simulink model "PID"  (R2017a)
settings: Solver=ode45  StartTime=0.0  StopTime=50  RelTol=1e-3  EnableMultiTasking=on
undefined symbols (not defined in the file): PID, thesis_lib
libraries: realtime_pacer_lib x1
settings Model: Creator=Waleed Niaz  LastModifiedBy=Waleed Niaz
settings DataIOCC: LimitDataPoints=on  SaveFormat=Array  SignalLoggingSaveFormat=ModelDataLogs
settings OptimizationCC: BooleanDataType=off
settings DebuggingCC: SaveWithParameterizedLinksMsg=none  UnderspecifiedInitializationDetection=Classic  MergeDetectMultiDrivingBlocksExec=none  SignalResolutionControl=TryResolveAllWithWarning  MultiTaskDSMMsg=warning  MultiTaskCondExecSysMsg=none
settings HardwareCC: TargetUnknown=on
settings ModelReferenceCC: PropagateSignalLabelsOutOfModel=off
settings GRTTargetCC: TargetLangStandard=C89/C90 (ANSI)  CombineOutputUpdateFcns=off  GRTInterface=on
settings ConfigComp: CovMetricSettings=dw  CovHtmlReporting=on  CovSaveCumulativeToWorkspaceVar=on  CovSaveSingleToWorkspaceVar=on  CovExternalEMLEnable=off

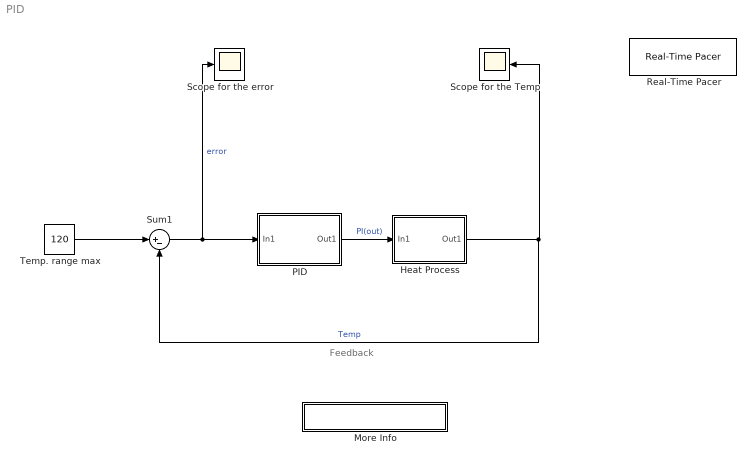
== system PID ==
  note: Feedback
  Heat Process : Subsystem  mask(Process){T2=120, T1=75, F1=4, V=6}
      mask prompts: T2 "Temperature of hot water"; T1 "Temperature of cold water"; F1 "Flow rate of cold water"; V "Volume of the tank"
      mask help: The values for the temperature should be expressed in either degree Rankine or Kelvin.
      mask Display: disp('PROCESS')
  More Info : Subsystem
      mask Display: disp('Click here more information')
  PID : Subsystem  AncestorBlock=thesis_lib/PID  mask(PID Controller (Zervin's block)){P=0.9, I=0.4, D=0}
      mask prompts: P "Proportional Gain, Kp"; I "Integral Gain, Ki"; D "Derivative Gain, Kd"
      mask help: This Block is a model of a PID controller
      mask Help: Enter a value for Kp, Ki, and Kd.
      mask Display:
      | disp('PID \n\n');
      | disp('Controller');
  Real-Time Pacer : realtime_pacer_lib/Real-Time Pacer  simTimePerRealTime=1
  Scope for the Temp : Scope
  Scope for the error : Scope
  Sum1 : Sum  Inputs=|+-
  Temp. range max : Constant  Value=120  VectorParams1D=off
  wires:
  Sum1/1 -> Scope for the error/1, PID/1(In1)  "error"
  PID/1(Out1) -> Heat Process/1(In1)  "PI(out)"
  Heat Process/1(Out1) -> Sum1/2, Scope for the Temp/1  "Temp"
  Temp. range max/1 -> Sum1/1

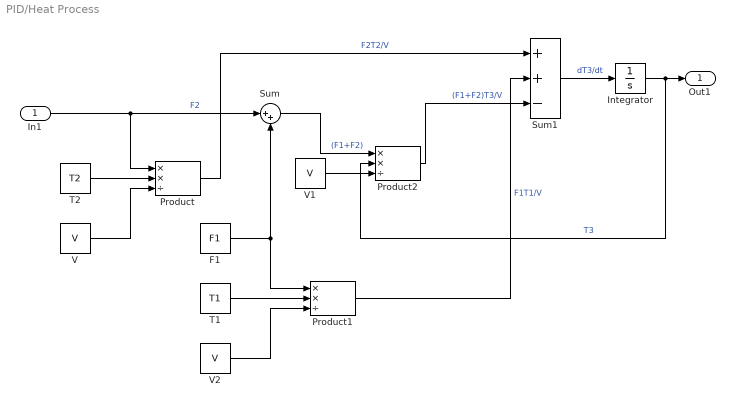
== system PID/Heat Process ==
  In1 : Inport
  F1 : Constant  Value=F1
  Integrator : Integrator  InitialCondition=T1
  Product : Product  Inputs=**/  SaturateOnIntegerOverflow=on  RndMeth=Zero  InputSameDT=on  OutDataTypeStr=Inherit: Same as first input
  Product1 : Product  Inputs=**/  SaturateOnIntegerOverflow=on  RndMeth=Zero  InputSameDT=on  OutDataTypeStr=Inherit: Same as first input
  Product2 : Product  Inputs=**/  SaturateOnIntegerOverflow=on  RndMeth=Zero  InputSameDT=on  OutDataTypeStr=Inherit: Same as first input
  Sum : Sum  Inputs=|++  SaturateOnIntegerOverflow=on  InputSameDT=on  OutDataTypeStr=Inherit: Same as first input
  Sum1 : Sum  Inputs=|++-  SaturateOnIntegerOverflow=on  InputSameDT=on  OutDataTypeStr=Inherit: Same as first input
  T1 : Constant  Value=T1
  T2 : Constant  Value=T2
  V : Constant  Value=V
  V1 : Constant  Value=V
  V2 : Constant  Value=V
  Out1 : Outport
  wires:
  In1/1 -> Product/1, Sum/1  "F2"
  V/1 -> Product/3
  F1/1 -> Product1/1, Sum/2
  T1/1 -> Product1/2
  V2/1 -> Product1/3
  V1/1 -> Product2/3
  Sum/1 -> Product2/1  "(F1+F2)"
  Product/1 -> Sum1/1  "F2T2/V"
  Product1/1 -> Sum1/2  "F1T1/V"
  Product2/1 -> Sum1/3  "(F1+F2)T3/V"
  Sum1/1 -> Integrator/1  "dT3/dt"
  Integrator/1 -> Product2/2, Out1/1  "T3"
  T2/1 -> Product/2

== system PID/More Info ==
  note: Before starting the simulation of the
      | system, the constant parameters of the system
      | must first be supplied to the model.
      | i.e the PI constant values
  note: Here are the parameters that needs to be specified:
  note: 1.) For the Temp. set point block, the Temperature set point or the desired
      | temperature.
      | 2.) For the PID controller block, the value of Kp, Ki and Kd.
      | 3.) For the process block, the Temperature of the incoming flows, the flowrate of the cold water and the volume of the tank.
      | 4.) Real time pacer uses the matlab pause and show the real time simulation in seconds.
      | 5.) Real time pacer library is not a built-in library we have to download it online.
      | 6.) If real time pacer block is not found then run again the file real_time_pacer.lib and add the block.
  note: The response or the result of the simulation can be viewed
      | by double-clicking the scope blocks.

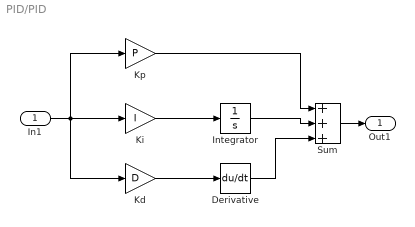
== system PID/PID ==
  In1 : Inport
  Derivative : Derivative
  Integrator : Integrator
  Kd : Gain  Gain=D  SaturateOnIntegerOverflow=on  OutDataTypeStr=Inherit: Same as input  ParamDataTypeStr=Inherit: Same as input
  Ki : Gain  Gain=I  SaturateOnIntegerOverflow=on  OutDataTypeStr=Inherit: Same as input  ParamDataTypeStr=Inherit: Same as input
  Kp : Gain  Gain=P  SaturateOnIntegerOverflow=on  OutDataTypeStr=Inherit: Same as input  ParamDataTypeStr=Inherit: Same as input
  Sum : Sum  Inputs=|+++  SaturateOnIntegerOverflow=on  InputSameDT=on  OutDataTypeStr=Inherit: Same as first input
  Out1 : Outport
  wires:
  Sum/1 -> Out1/1
  Derivative/1 -> Sum/3
  Integrator/1 -> Sum/2
  Kp/1 -> Sum/1
  Kd/1 -> Derivative/1
  Ki/1 -> Integrator/1
  In1/1 -> Ki/1, Kp/1, Kd/1
